simulink model "delay_pos_pos"  (R2020b)
settings: Solver=FixedStepAuto  StartTime=0.0  StopTime=30  FixedStep=Ts  MinStep=1e-5  RelTol=1e-5
undefined symbols (not defined in the file): A, A_int, B, b, Be, Bh_i, Bm, Bs, C, delayT, Dh, DiscIntNeverNeededParam, Discrete, Dm, Ds, Fc, Fip, Jh_i, Ke, Kh, Kh_i, Km, Ks, Mm, Ms, posNoiseVariance, R, Time, Ts, xe
libraries: simulink x2, ctrlSharedLib x2, cstblocks x1
settings Model: Creator=simon  LastModifiedBy=simon
settings SolverCC: AlgebraicLoopSolver=LineSearch

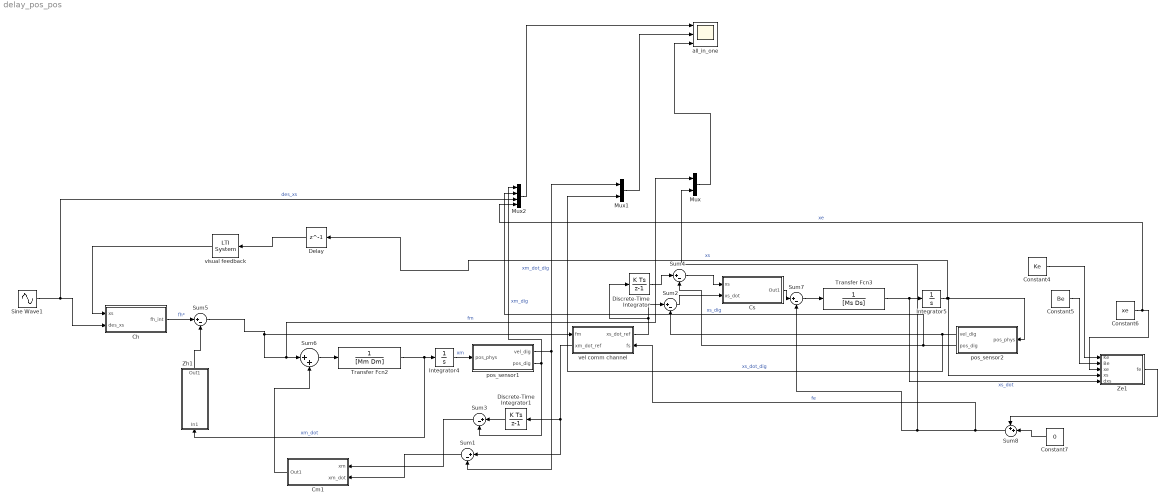
== system delay_pos_pos ==
  Ch : Subsystem
  Cm1 : Subsystem
  Constant4 : Constant  Value=Ke
  Constant5 : Constant  Value=Be
  Constant6 : Constant  Value=xe
  Constant7 : Constant  Value=0
  Cs : Subsystem
  Delay : Delay  DelayLength=1  SampleTime=Ts
  Discrete-Time Integrator : DiscreteIntegrator  SampleTime=-1  ICPrevOutput=DiscIntNeverNeededParam  ICPrevScaledInput=DiscIntNeverNeededParam
  Discrete-Time Integrator1 : DiscreteIntegrator  SampleTime=-1  ICPrevOutput=DiscIntNeverNeededParam  ICPrevScaledInput=DiscIntNeverNeededParam
  Integrator4 : Integrator
  Integrator5 : Integrator
  Mux : Mux  Inputs=2
  Mux1 : Mux  Inputs=2
  Mux2 : Mux
  Sine Wave1 : Sin  Amplitude=A_int  Frequency=Fc  SampleTime=0
  Sum{1..5,7} (6 alike) : Sum  Inputs=|+-
  Sum6 : Sum  Inputs=|++
  Sum8 : Sum  Inputs=++|
  Transfer Fcn2 : TransferFcn  Denominator=[Mm Dm]
  Transfer Fcn3 : TransferFcn  Denominator=[Ms Ds]
  Ze1 : MATLAB Function  TreatAsAtomicUnit=on
  Zh1 : Subsystem
  all_in_one : Scope  NumInputPorts=3
  pos_sensor1 : Subsystem
  pos_sensor2 : Subsystem
  vel comm channel : Subsystem
      settings: PortSchema="{\"entries\":[{\"content\":{\"sides\":[{\"content\":{\"connectorIds\":[\"In1\",\"Out2\"]},\"type\":\"ConnectorPlacement.EquallySpacedRectSide\",\"uuid\":\"087ef83c-4534-4f3f-ad60-ce2423e06c57\"},{\"content\":{\"connectorIds\":[\"Out1\",\"In2\"],\"side\":\"RIGHT\"},\"type\":\"ConnectorPlacement.EquallySpacedRectSide\",\"uuid\":\"019153fa-edd0-4560-9bcd-9bc8080d4b6a\"},{\"content\":{\"connectorIds\":[],\"side\":\"TOP\"},\"type\":\"ConnectorPlacement.EquallySpacedRectSide\",\"uuid\":\"d3514247-cab7-4f3c-b49a-6c3bfe2b0cf3\"},{\"content\":{\"connectorIds\":[],\"side\":\"HIDDEN\"},\"type\":\"ConnectorPlacement.EquallySpacedRectSide\",\"uuid\":\"fe58816e-1afb-4836-94a8-7d74059b88c3\"}]},\"type\":\"ConnectorPlacement.EquallySpacedConnector\",\"uuid\":\"0c1d979d-cda7-4b3e-b96e-a73b026bb6ed\"}],\"packageUris\":[\"http://schema.mathworks.com/mf0/Connector/R2020b\"],\"version\":\"1.0\"}"
  visual feedback : cstblocks/LTI System  sys=1  IC=[]
  wires:
  Integrator5/1 -> Delay/1, pos_sensor2/1(pos_phys), Ze1/4(xs)  "xs"
  Ch/1(fh_int) -> Sum5/1  "fh*"
  Sum6/1 -> Transfer Fcn2/1
  Sum5/1 -> vel comm channel/1(fm), Mux/1, Sum6/1  "fm"
  Zh1/1(Out1) -> Sum5/2
  Constant5/1 -> Ze1/2(Be)
  Constant7/1 -> Sum8/2
  Constant6/1 -> Mux2/4, Ze1/3(xe)  "xe"
  Integrator4/1 -> pos_sensor1/1(pos_phys)  "xm"
  Transfer Fcn2/1 -> Zh1/1(In1), Integrator4/1  "xm_dot"
  Ze1/1(fe) -> Sum8/1
  Constant4/1 -> Ze1/1(Ke)
  pos_sensor1/1(vel_dig) -> Mux1/1, Sum1/2  "xm_dot_dig"
  Transfer Fcn3/1 -> Ze1/5(dxs), Integrator5/1  "xs_dot"
  Sum7/1 -> Transfer Fcn3/1
  Sum8/1 -> vel comm channel/2(fs), Mux/2, Sum7/2  "fe"
  Sine Wave1/1 -> Mux2/3, Ch/2(des_xs)  "des_xs"
  Delay/1 -> visual feedback/1
  visual feedback/1 -> Ch/1(xs)
  Sum2/1 -> Cs/2(xs_dot)
  Sum4/1 -> Cs/1(xs)
  vel comm channel/1(xs_dot_ref) -> Discrete-Time Integrator/1, Sum2/1
  Cs/1(Out1) -> Sum7/1
  Cm1/1(Out1) -> Sum6/2
  vel comm channel/2(xm_dot_ref) -> Discrete-Time Integrator1/1, Sum1/1
  Sum1/1 -> Cm1/2(xm_dot)
  Discrete-Time Integrator1/1 -> Sum3/1
  pos_sensor1/2(pos_dig) -> Mux2/1, Sum3/2  "xm_dig"
  Sum3/1 -> Cm1/1(xm)
  Discrete-Time Integrator/1 -> Sum4/1
  pos_sensor2/2(pos_dig) -> Mux2/2, Sum4/2  "xs_dig"
  pos_sensor2/1(vel_dig) -> Mux1/2, Sum2/2  "xs_dot_dig"
  Mux/1 -> all_in_one/3
  Mux1/1 -> all_in_one/2
  Mux2/1 -> all_in_one/1

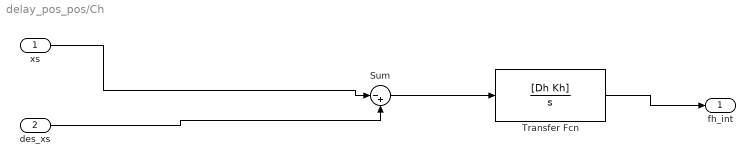
== system delay_pos_pos/Ch ==
  xs : Inport
  des_xs : Inport  Port=2
  Sum : Sum  Inputs=|-+
  Transfer Fcn : TransferFcn  Numerator=[Dh Kh]  Denominator=[1 0]
  fh_int : Outport
  wires:
  xs/1 -> Sum/1
  des_xs/1 -> Sum/2
  Sum/1 -> Transfer Fcn/1
  Transfer Fcn/1 -> fh_int/1

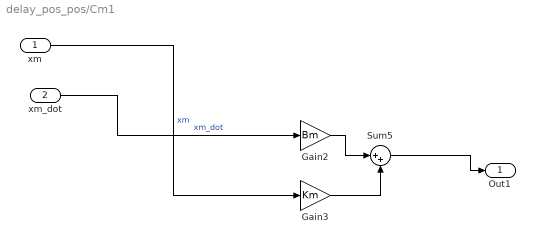
== system delay_pos_pos/Cm1 ==
  xm : Inport
  xm_dot : Inport  Port=2
  Gain2 : Gain  Gain=Bm
  Gain3 : Gain  Gain=Km
  Sum5 : Sum  Inputs=|++
  Out1 : Outport
  wires:
  xm/1 -> Gain3/1  "xm"
  Gain2/1 -> Sum5/1
  xm_dot/1 -> Gain2/1  "xm_dot"
  Gain3/1 -> Sum5/2
  Sum5/1 -> Out1/1

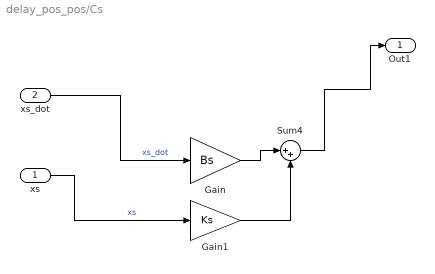
== system delay_pos_pos/Cs ==
  xs : Inport
  xs_dot : Inport  Port=2
  Gain : Gain  Gain=Bs
  Gain1 : Gain  Gain=Ks
  Sum4 : Sum  Inputs=|++
  Out1 : Outport
  wires:
  Gain1/1 -> Sum4/2
  Sum4/1 -> Out1/1
  xs_dot/1 -> Gain/1  "xs_dot"
  Gain/1 -> Sum4/1
  xs/1 -> Gain1/1  "xs"

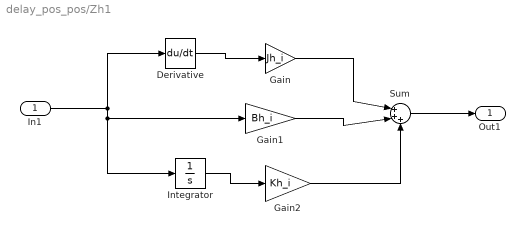
== system delay_pos_pos/Zh1 ==
  In1 : Inport
  Derivative : Derivative
  Gain : Gain  Gain=Jh_i
  Gain1 : Gain  Gain=Bh_i
  Gain2 : Gain  Gain=Kh_i
  Integrator : Integrator
  Sum : Sum  Inputs=|+++
  Out1 : Outport
  wires:
  Derivative/1 -> Gain/1
  Integrator/1 -> Gain2/1
  In1/1 -> Integrator/1, Gain1/1, Derivative/1
  Gain/1 -> Sum/1
  Gain1/1 -> Sum/2
  Gain2/1 -> Sum/3
  Sum/1 -> Out1/1

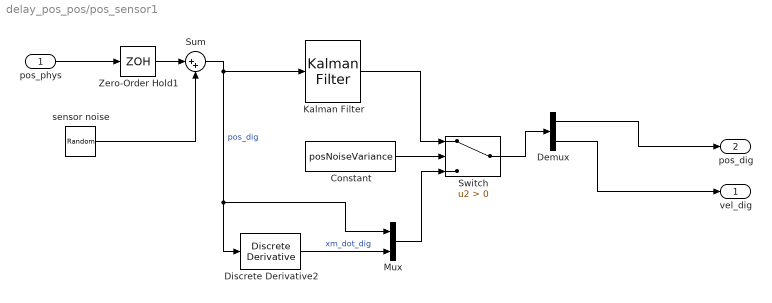
== system delay_pos_pos/pos_sensor1 ==
  pos_phys : Inport
  Constant : Constant  Value=posNoiseVariance
  Demux : Demux  Outputs=2
  Discrete Derivative2 : simulink/Discrete/Discrete Derivative  gainval=1.0  ICPrevScaledInput=0.0  OutMin=[]  OutMax=[]  OutDataType=fixdt(1, 16)  OutScaling=2^-10  DoSatur=off
  Kalman Filter : ctrlSharedLib/Kalman Filter  TimeDomain=Discrete-Time  UseCurrentEstimator=on  ModelSource=Individual A, B, C, D matrices  ModelSourceVariable=ss(0.95,1,1,0,1)  A=A  B=B  C=C  D=0  NumberOfStates=2  NumberOfInputs=1  NumberOfOutputs=1  InitialEstimateSource=Dialog  X0=0  P0=10  UseK=off  UseGH=off  NumberOfProcessNoiseInputs=1  G=1  TimeInvariantG=on  H=0  TimeInvariantH=on  Q=Q_m  TimeInvariantQ=on  R=R  TimeInvariantR=on  N=0  TimeInvariantN=on  AddInputPort=off  AddEnablePort=off  OutputEstimatedY=off  OutputP=off  Ts=Ts
  Mux : Mux  Inputs=2
  Sum : Sum  Inputs=|++
  Switch : Switch  Criteria=u2 > Threshold
  Zero-Order Hold1 : ZeroOrderHold  SampleTime=Ts
  sensor noise : RandomNumber  Variance=posNoiseVariance  SampleTime=Ts
  vel_dig : Outport
  pos_dig : Outport  Port=2
  wires:
  pos_phys/1 -> Zero-Order Hold1/1
  Zero-Order Hold1/1 -> Sum/1
  sensor noise/1 -> Sum/2
  Kalman Filter/1 -> Switch/1
  Sum/1 -> Mux/1, Discrete Derivative2/1, Kalman Filter/1  "pos_dig"
  Constant/1 -> Switch/2
  Mux/1 -> Switch/3
  Discrete Derivative2/1 -> Mux/2  "xm_dot_dig"
  Switch/1 -> Demux/1
  Demux/1 -> pos_dig/1
  Demux/2 -> vel_dig/1

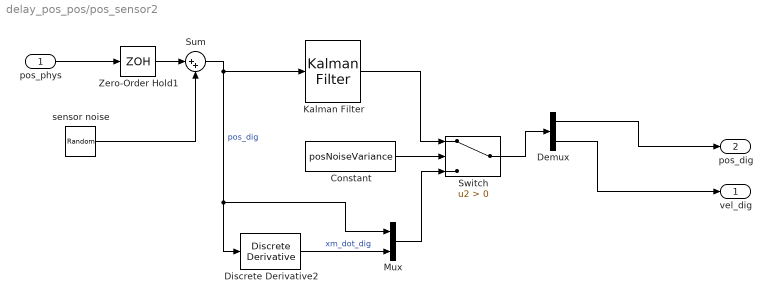
== system delay_pos_pos/pos_sensor2 ==
  pos_phys : Inport
  Constant : Constant  Value=posNoiseVariance
  Demux : Demux  Outputs=2
  Discrete Derivative2 : simulink/Discrete/Discrete Derivative  gainval=1.0  ICPrevScaledInput=0.0  OutMin=[]  OutMax=[]  OutDataType=fixdt(1, 16)  OutScaling=2^-10  DoSatur=off
  Kalman Filter : ctrlSharedLib/Kalman Filter  TimeDomain=Discrete-Time  UseCurrentEstimator=on  ModelSource=Individual A, B, C, D matrices  ModelSourceVariable=ss(0.95,1,1,0,1)  A=A  B=B  C=C  D=0  NumberOfStates=2  NumberOfInputs=1  NumberOfOutputs=1  InitialEstimateSource=Dialog  X0=0  P0=10  UseK=off  UseGH=off  NumberOfProcessNoiseInputs=1  G=1  TimeInvariantG=on  H=0  TimeInvariantH=on  Q=Q_m  TimeInvariantQ=on  R=R  TimeInvariantR=on  N=0  TimeInvariantN=on  AddInputPort=off  AddEnablePort=off  OutputEstimatedY=off  OutputP=off  Ts=Ts
  Mux : Mux  Inputs=2
  Sum : Sum  Inputs=|++
  Switch : Switch  Criteria=u2 > Threshold
  Zero-Order Hold1 : ZeroOrderHold  SampleTime=Ts
  sensor noise : RandomNumber  Variance=posNoiseVariance  SampleTime=Ts
  vel_dig : Outport
  pos_dig : Outport  Port=2
  wires:
  pos_phys/1 -> Zero-Order Hold1/1
  Zero-Order Hold1/1 -> Sum/1
  sensor noise/1 -> Sum/2
  Kalman Filter/1 -> Switch/1
  Sum/1 -> Mux/1, Discrete Derivative2/1, Kalman Filter/1  "pos_dig"
  Constant/1 -> Switch/2
  Mux/1 -> Switch/3
  Discrete Derivative2/1 -> Mux/2  "xm_dot_dig"
  Switch/1 -> Demux/1
  Demux/1 -> pos_dig/1
  Demux/2 -> vel_dig/1

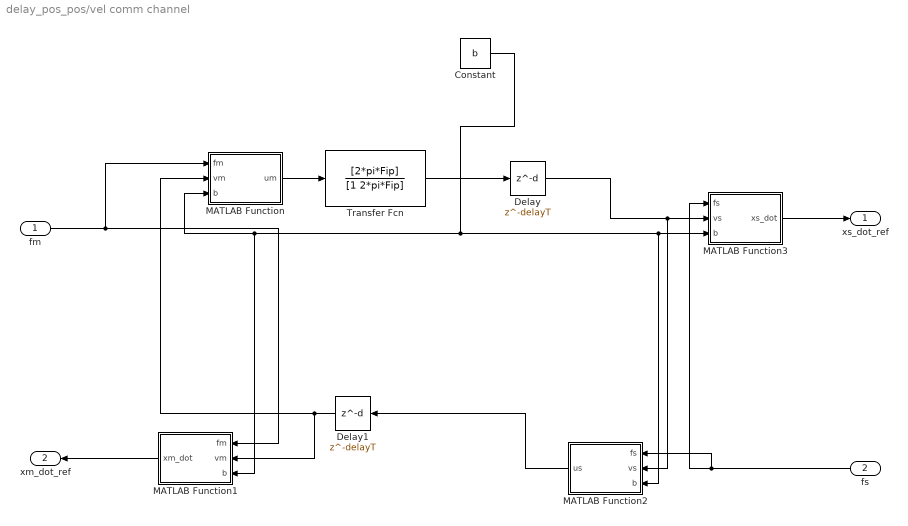
== system delay_pos_pos/vel comm channel ==
  fm : Inport
  fs : Inport  Port=2
  Constant : Constant  Value=b
  Delay : Delay  DelayLength=delayT  SampleTime=Ts
  Delay1 : Delay  DelayLength=delayT  SampleTime=Ts
  MATLAB Function : MATLAB Function  TreatAsAtomicUnit=on
  MATLAB Function1 : MATLAB Function  TreatAsAtomicUnit=on
  MATLAB Function2 : MATLAB Function  TreatAsAtomicUnit=on
  MATLAB Function3 : MATLAB Function  TreatAsAtomicUnit=on
  Transfer Fcn : TransferFcn  Numerator=[2*pi*Fip]  Denominator=[1 2*pi*Fip]
  xs_dot_ref : Outport
  xm_dot_ref : Outport  Port=2
  wires:
  Constant/1 -> MATLAB Function1/3(b), MATLAB Function/3(b), MATLAB Function2/3(b), MATLAB Function3/3(b)
  Delay/1 -> MATLAB Function2/2(vs), MATLAB Function3/2(vs)
  Delay1/1 -> MATLAB Function/2(vm), MATLAB Function1/2(vm)
  MATLAB Function/1(um) -> Transfer Fcn/1
  MATLAB Function2/1(us) -> Delay1/1
  fm/1 -> MATLAB Function1/1(fm), MATLAB Function/1(fm)
  fs/1 -> MATLAB Function2/1(fs), MATLAB Function3/1(fs)
  MATLAB Function3/1(xs_dot) -> xs_dot_ref/1
  MATLAB Function1/1(xm_dot) -> xm_dot_ref/1
  Transfer Fcn/1 -> Delay/1

== matlab function delay_pos_pos/vel comm channel/MATLAB Function ==
  data: fm input; um output; vm input; b input
function um = fcn(fm, vm, b)

um = sqrt(2/b)*fm-vm;

== matlab function delay_pos_pos/vel comm channel/MATLAB Function1 ==
  data: fm input; xm_dot output; vm input; b input
function xm_dot = fcn(fm, vm, b)

xm_dot = (1/b)*(fm-sqrt(2*b)*vm);

== matlab function delay_pos_pos/vel comm channel/MATLAB Function2 ==
  data: fs input; us output; vs input; b input
function us = fcn(fs, vs, b)

us = sqrt(2/b)*fs-vs;

== matlab function delay_pos_pos/vel comm channel/MATLAB Function3 ==
  data: fs input; xs_dot output; vs input; b input
function xs_dot = fcn(fs, vs, b)

xs_dot = -(1/b)*(fs - sqrt(2*b)*vs);

== matlab function delay_pos_pos/Ze1 ==
  data: Ke input; fe output; Be input; xe input; xs input; dxs input
function fe = env(Ke, Be, xe, xs, dxs)
    if xs > xe
        fe = Ke*(xs-xe)+Be*max(dxs, 0);
    else
        fe = 0;
    end
